simulink model "lab6_simulink"  (R2024a)
settings: Solver=VariableStepAuto  StartTime=0.0  StopTime=1  RelTol=1e-3
libraries: dspfdesign x2, dspsrcs4 x2
settings Model: Creator=pulley  LastModifiedBy=pulley

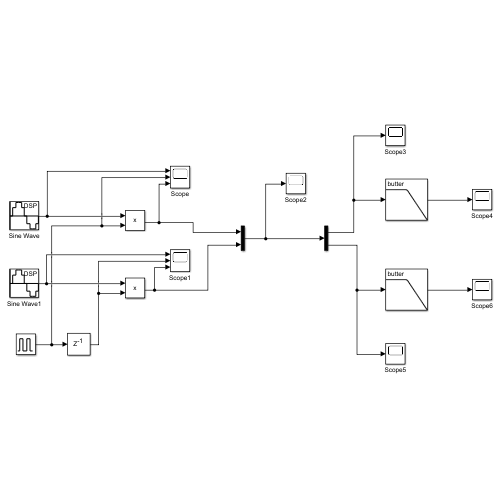
[thumbnail: Simulink's stored preview of the top-level diagram]
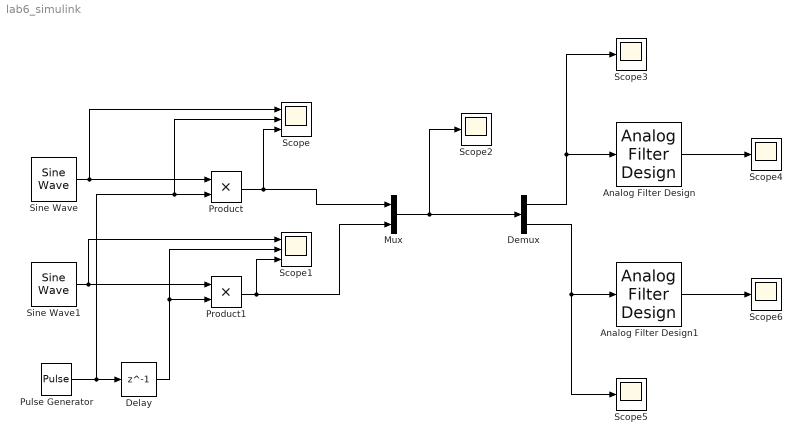
== system lab6_simulink ==
  Analog Filter Design : dspfdesign/Analog Filter Design  method=Butterworth  filttype=Lowpass  N=8  Wlo=2*pi*10  Whi=80  Rp=2  Rs=40
  Analog Filter Design1 : dspfdesign/Analog Filter Design  method=Butterworth  filttype=Lowpass  N=8  Wlo=2*pi*20  Whi=80  Rp=2  Rs=40
  Delay : Delay  DelayLength=1  SampleTime=0.001
  Demux : Demux  Outputs=2
  Mux : Mux  Inputs=2
  Product : Product
  Product1 : Product
  Pulse Generator : DiscretePulseGenerator  PulseType=Time based  Period=0.01  PulseWidth=5
  Scope : Scope  NumInputPorts=3
  Scope1 : Scope  NumInputPorts=3
  Scope{2..6} (5 alike) : Scope
  Sine Wave : dspsrcs4/Sine Wave  Amplitude=1  Frequency=2*pi*10  Phase=0  SampleMode=Discrete  OutComplex=Real  CompMethod=Trigonometric fcn  TableSize=Speed  SampleTime=0.001  SamplesPerFrame=1  ResetState=Restart at time zero  OutputFrames=off  dataType=double  wordLen=16  udDataType=sfix(16)  fracBitsMode=Best precision  numFracBits=15  OutDataTypeStr=double  LastOutDataTypeStr=double
  Sine Wave1 : dspsrcs4/Sine Wave  Amplitude=2  Frequency=2*pi*20  Phase=0  SampleMode=Discrete  OutComplex=Real  CompMethod=Trigonometric fcn  TableSize=Speed  SampleTime=0.001  SamplesPerFrame=1  ResetState=Restart at time zero  OutputFrames=off  dataType=double  wordLen=16  udDataType=sfix(16)  fracBitsMode=Best precision  numFracBits=15  OutDataTypeStr=double  LastOutDataTypeStr=double
  wires:
  Sine Wave/1 -> Scope/1, Product/1
  Sine Wave1/1 -> Scope1/1, Product1/1
  Pulse Generator/1 -> Scope/2, Product/2, Delay/1
  Delay/1 -> Product1/2, Scope1/2
  Product/1 -> Mux/1, Scope/3
  Product1/1 -> Scope1/3, Mux/2
  Mux/1 -> Demux/1, Scope2/1
  Demux/1 -> Scope3/1, Analog Filter Design/1
  Demux/2 -> Analog Filter Design1/1, Scope5/1
  Analog Filter Design/1 -> Scope4/1
  Analog Filter Design1/1 -> Scope6/1
